simulink model "black_ice_lidar_geometry"  (R2024a)
settings: Solver=FixedStepDiscrete  StartTime=0  StopTime=0  FixedStep=1  RelTol=1e-3
model workspace (MAT data in the model file):
  H_m = 1.6
  t_m = 0.03
  theta_deg = 0
Description:
  | blackice_checkpoint01_generated: Level 0 simulation-only; theta from road normal; DA=H/cos(theta), DI=(H-t)/cos(theta). Invalid ranges are NaN. Generated by build_geometry_simulink_model.

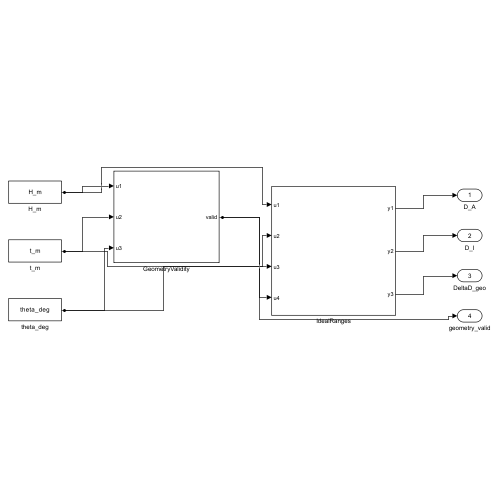
[thumbnail: Simulink's stored preview of the top-level diagram]
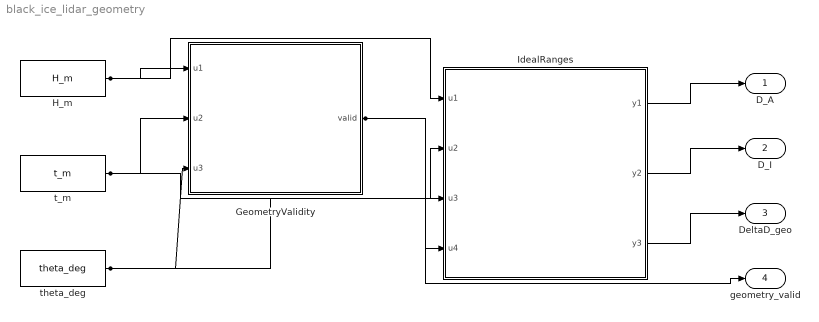
== system black_ice_lidar_geometry ==
  GeometryValidity : Subsystem
  H_m : Constant  Value=H_m
  IdealRanges : Subsystem
  t_m : Constant  Value=t_m
  theta_deg : Constant  Value=theta_deg
  D_A : Outport
  D_I : Outport  Port=2
  DeltaD_geo : Outport  Port=3
  geometry_valid : Outport  Port=4
  wires:
  H_m/1 -> GeometryValidity/1(u1), IdealRanges/1(u1)
  t_m/1 -> GeometryValidity/2(u2), IdealRanges/2(u2)
  theta_deg/1 -> GeometryValidity/3(u3), IdealRanges/3(u3)
  GeometryValidity/1(valid) -> IdealRanges/4(u4), geometry_valid/1
  IdealRanges/1(y1) -> D_A/1
  IdealRanges/2(y2) -> D_I/1
  IdealRanges/3(y3) -> DeltaD_geo/1

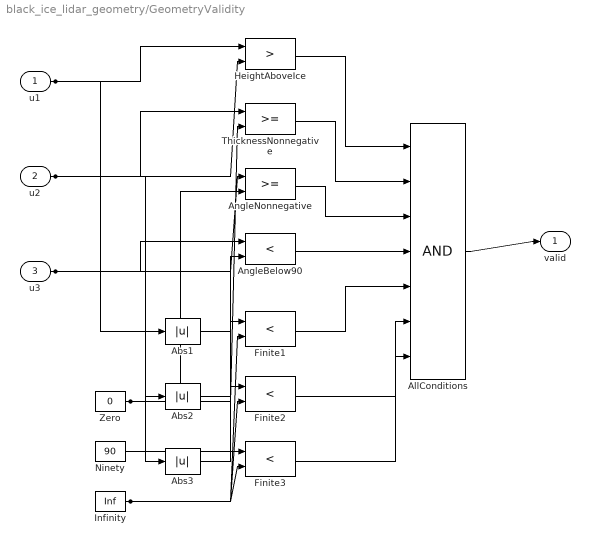
== system black_ice_lidar_geometry/GeometryValidity ==
  u1 : Inport
  u2 : Inport  Port=2
  u3 : Inport  Port=3
  Abs1 : Abs  SaturateOnIntegerOverflow=off
  Abs2 : Abs  SaturateOnIntegerOverflow=off
  Abs3 : Abs  SaturateOnIntegerOverflow=off
  AllConditions : Logic  Inputs=7  AllPortsSameDT=off  OutDataTypeStr=boolean
  AngleBelow90 : RelationalOperator  Operator=<  OutDataTypeStr=boolean  RndMeth=Simplest  InputSameDT=off
  AngleNonnegative : RelationalOperator  OutDataTypeStr=boolean  RndMeth=Simplest  InputSameDT=off
  Finite1 : RelationalOperator  Operator=<  OutDataTypeStr=boolean  RndMeth=Simplest  InputSameDT=off
  Finite2 : RelationalOperator  Operator=<  OutDataTypeStr=boolean  RndMeth=Simplest  InputSameDT=off
  Finite3 : RelationalOperator  Operator=<  OutDataTypeStr=boolean  RndMeth=Simplest  InputSameDT=off
  HeightAboveIce : RelationalOperator  Operator=>  OutDataTypeStr=boolean  RndMeth=Simplest  InputSameDT=off
  Infinity : Constant  Value=Inf
  Ninety : Constant  Value=90
  ThicknessNonnegative : RelationalOperator  OutDataTypeStr=boolean  RndMeth=Simplest  InputSameDT=off
  Zero : Constant  Value=0
  valid : Outport
  wires:
  u1/1 -> HeightAboveIce/1, Abs1/1
  u2/1 -> HeightAboveIce/2, ThicknessNonnegative/1, Abs2/1
  Zero/1 -> ThicknessNonnegative/2, AngleNonnegative/2
  u3/1 -> AngleNonnegative/1, AngleBelow90/1, Abs3/1
  Ninety/1 -> AngleBelow90/2
  Abs1/1 -> Finite1/1
  Infinity/1 -> Finite1/2, Finite2/2, Finite3/2
  Abs2/1 -> Finite2/1
  Abs3/1 -> Finite3/1
  HeightAboveIce/1 -> AllConditions/1
  ThicknessNonnegative/1 -> AllConditions/2
  AngleNonnegative/1 -> AllConditions/3
  AngleBelow90/1 -> AllConditions/4
  Finite1/1 -> AllConditions/5
  Finite2/1 -> AllConditions/6
  Finite3/1 -> AllConditions/7
  AllConditions/1 -> valid/1

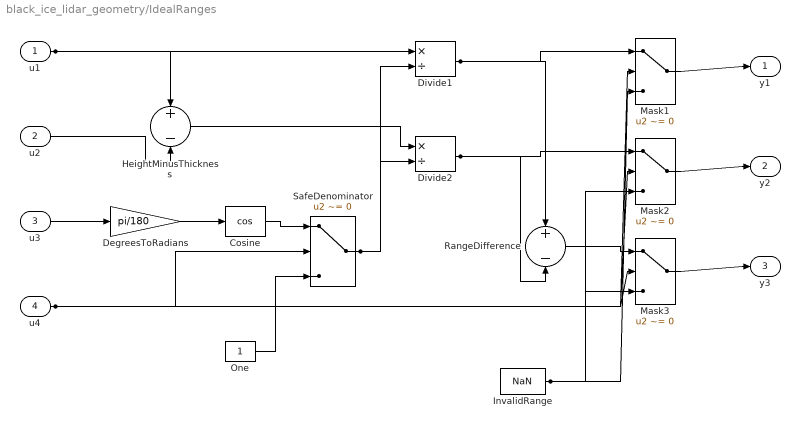
== system black_ice_lidar_geometry/IdealRanges ==
  u1 : Inport
  u2 : Inport  Port=2
  u3 : Inport  Port=3
  u4 : Inport  Port=4
  Cosine : Trigonometry  Operator=cos
  DegreesToRadians : Gain  Gain=pi/180
  Divide1 : Product  Inputs=*/
  Divide2 : Product  Inputs=*/
  HeightMinusThickness : Sum  Inputs=+-
  InvalidRange : Constant  Value=NaN
  Mask1 : Switch  Criteria=u2 ~= 0  SaturateOnIntegerOverflow=off  InputSameDT=off
  Mask2 : Switch  Criteria=u2 ~= 0  SaturateOnIntegerOverflow=off  InputSameDT=off
  Mask3 : Switch  Criteria=u2 ~= 0  SaturateOnIntegerOverflow=off  InputSameDT=off
  One : Constant
  RangeDifference : Sum  Inputs=+-
  SafeDenominator : Switch  Criteria=u2 ~= 0  SaturateOnIntegerOverflow=off  InputSameDT=off
  y1 : Outport
  y2 : Outport  Port=2
  y3 : Outport  Port=3
  wires:
  u3/1 -> DegreesToRadians/1
  DegreesToRadians/1 -> Cosine/1
  Cosine/1 -> SafeDenominator/1
  u4/1 -> SafeDenominator/2, Mask1/2, Mask2/2, Mask3/2
  One/1 -> SafeDenominator/3
  u1/1 -> HeightMinusThickness/1, Divide1/1
  u2/1 -> HeightMinusThickness/2
  SafeDenominator/1 -> Divide1/2, Divide2/2
  HeightMinusThickness/1 -> Divide2/1
  Divide1/1 -> RangeDifference/1, Mask1/1
  Divide2/1 -> RangeDifference/2, Mask2/1
  InvalidRange/1 -> Mask1/3, Mask2/3, Mask3/3
  Mask1/1 -> y1/1
  Mask2/1 -> y2/1
  RangeDifference/1 -> Mask3/1
  Mask3/1 -> y3/1
